simulink model "TST_StSys_StrtRmp"  (R2016b)
settings: Solver=FixedStepDiscrete  StartTime=0.0  StopTime=simTime  FixedStep=sampleTime  RelTol=1e-3
values from neighbouring files (symbols this model uses):
  testCase = 1    [initTST_StSys_StrtRmp_001.m]
libraries: simulink x3, UnitTest_Lib x1
settings Model: Creator=zhengjinyan  LastModifiedBy=zhengjinyan
settings DebuggingCC: SignalRangeChecking=error

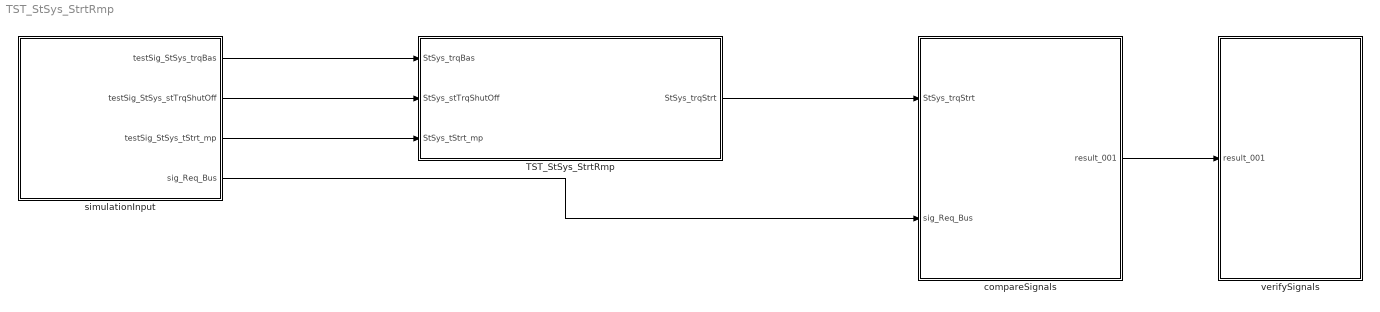
== system TST_StSys_StrtRmp ==
  TST_StSys_StrtRmp : Subsystem
  compareSignals : Subsystem
  simulationInput : Subsystem
  verifySignals : Subsystem
  wires:
  simulationInput/1(testSig_StSys_trqBas) -> TST_StSys_StrtRmp/1(StSys_trqBas)
  simulationInput/2(testSig_StSys_stTrqShutOff) -> TST_StSys_StrtRmp/2(StSys_stTrqShutOff)
  simulationInput/3(testSig_StSys_tStrt_mp) -> TST_StSys_StrtRmp/3(StSys_tStrt_mp)
  TST_StSys_StrtRmp/1(StSys_trqStrt) -> compareSignals/1(StSys_trqStrt)
  simulationInput/4(sig_Req_Bus) -> compareSignals/2(sig_Req_Bus)
  compareSignals/1(result_001) -> verifySignals/1(result_001)

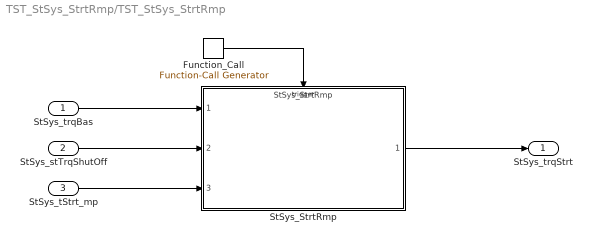
== system TST_StSys_StrtRmp/TST_StSys_StrtRmp ==
  StSys_trqBas : Inport
  StSys_stTrqShutOff : Inport  Port=2
  StSys_tStrt_mp : Inport  Port=3
  Function_Call : simulink/Ports & Subsystems/Function-Call Generator  sample_time=sampleTime  numberOfIterations=1
  StSys_StrtRmp : ModelReference  ModelNameDialog=StSys_StrtRmp  SimulationMode=Normal  ModelReferenceVersion=1.51  TriggerPortName=function  TriggerPortTriggerType=function-call  TriggerPortStatesWhenEnabling=held
  StSys_trqStrt : Outport
  wires:
  Function_Call/1 -> StSys_StrtRmp/Trigger
  StSys_trqBas/1 -> StSys_StrtRmp/1
  StSys_stTrqShutOff/1 -> StSys_StrtRmp/2
  StSys_tStrt_mp/1 -> StSys_StrtRmp/3
  StSys_StrtRmp/1 -> StSys_trqStrt/1

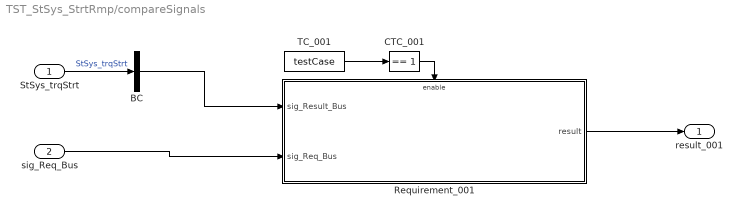
== system TST_StSys_StrtRmp/compareSignals ==
  StSys_trqStrt : Inport
  sig_Req_Bus : Inport  Port=2
  BC : BusCreator  Inputs=1
  CTC_001 : simulink/Logic and Bit Operations/Compare To Constant  relop===  const=1  OutDataTypeStr=boolean
  Requirement_001 : Subsystem
  TC_001 : Constant  Value=testCase
  result_001 : Outport
  wires:
  StSys_trqStrt/1 -> BC/1  "StSys_trqStrt"
  TC_001/1 -> CTC_001/1
  CTC_001/1 -> Requirement_001/Enable
  sig_Req_Bus/1 -> Requirement_001/2(sig_Req_Bus)
  BC/1 -> Requirement_001/1(sig_Result_Bus)
  Requirement_001/1(result) -> result_001/1

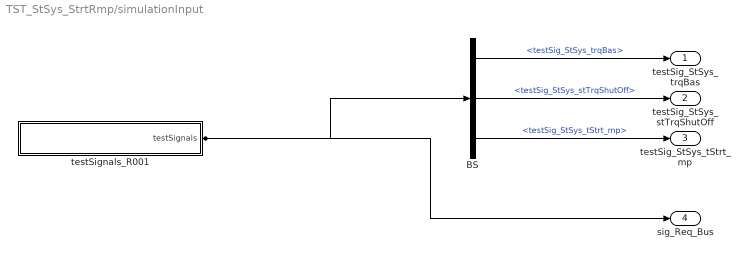
== system TST_StSys_StrtRmp/simulationInput ==
  BS : BusSelector  OutputSignals=testSig_StSys_trqBas,testSig_StSys_stTrqShutOff,testSig_StSys_tStrt_mp
  testSignals_R001 : Subsystem
  testSig_StSys_trqBas : Outport
  testSig_StSys_stTrqShutOff : Outport  Port=2
  testSig_StSys_tStrt_mp : Outport  Port=3
  sig_Req_Bus : Outport  Port=4
  wires:
  BS/1 -> testSig_StSys_trqBas/1  "<testSig_StSys_trqBas>"
  BS/2 -> testSig_StSys_stTrqShutOff/1  "<testSig_StSys_stTrqShutOff>"
  BS/3 -> testSig_StSys_tStrt_mp/1  "<testSig_StSys_tStrt_mp>"
  testSignals_R001/1(testSignals) -> BS/1, sig_Req_Bus/1

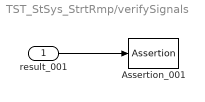
== system TST_StSys_StrtRmp/verifySignals ==
  result_001 : Inport
  Assertion_001 : Assertion  Enabled=off
  wires:
  result_001/1 -> Assertion_001/1

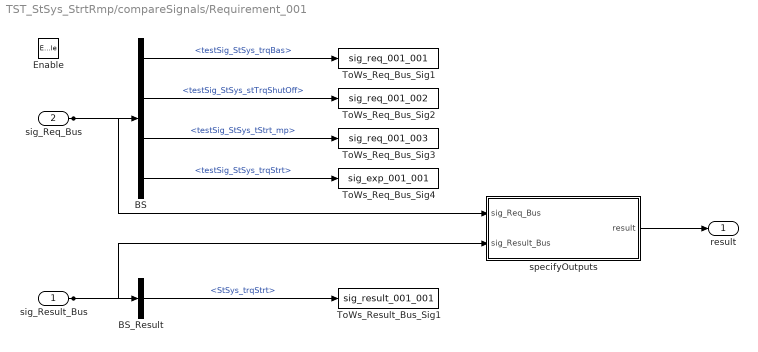
== system TST_StSys_StrtRmp/compareSignals/Requirement_001 ==
  sig_Result_Bus : Inport
  sig_Req_Bus : Inport  Port=2
  Enable : EnablePort
  BS : BusSelector  OutputSignals=testSig_StSys_trqBas,testSig_StSys_stTrqShutOff,testSig_StSys_tStrt_mp,testSig_StSys_trqStrt
  BS_Result : BusSelector  OutputSignals=StSys_trqStrt
  ToWs_Req_Bus_Sig1 : ToWorkspace  VariableName=sig_req_001_001  SaveFormat=Structure With Time
  ToWs_Req_Bus_Sig2 : ToWorkspace  VariableName=sig_req_001_002  SaveFormat=Structure With Time
  ToWs_Req_Bus_Sig3 : ToWorkspace  VariableName=sig_req_001_003  SaveFormat=Structure With Time
  ToWs_Req_Bus_Sig4 : ToWorkspace  VariableName=sig_exp_001_001  SaveFormat=Structure With Time
  ToWs_Result_Bus_Sig1 : ToWorkspace  VariableName=sig_result_001_001  SaveFormat=Structure With Time
  specifyOutputs : Subsystem
  result : Outport
  wires:
  sig_Req_Bus/1 -> BS/1, specifyOutputs/1(sig_Req_Bus)
  BS/1 -> ToWs_Req_Bus_Sig1/1  "<testSig_StSys_trqBas>"
  BS/2 -> ToWs_Req_Bus_Sig2/1  "<testSig_StSys_stTrqShutOff>"
  BS/3 -> ToWs_Req_Bus_Sig3/1  "<testSig_StSys_tStrt_mp>"
  BS/4 -> ToWs_Req_Bus_Sig4/1  "<testSig_StSys_trqStrt>"
  sig_Result_Bus/1 -> BS_Result/1, specifyOutputs/2(sig_Result_Bus)
  BS_Result/1 -> ToWs_Result_Bus_Sig1/1  "<StSys_trqStrt>"
  specifyOutputs/1(result) -> result/1

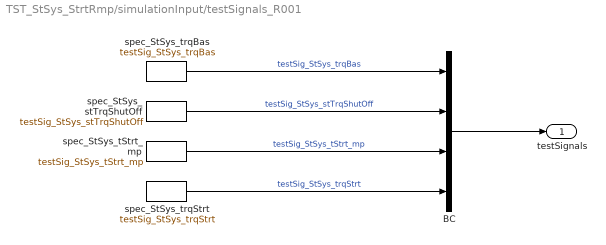
== system TST_StSys_StrtRmp/simulationInput/testSignals_R001 ==
  BC : BusCreator  Inputs=4
  spec_StSys_stTrqShutOff : FromWorkspace  VariableName=testSig_StSys_stTrqShutOff  Interpolate=off  OutputAfterFinalValue=Holding final value
  spec_StSys_tStrt_mp : FromWorkspace  VariableName=testSig_StSys_tStrt_mp  Interpolate=off  OutputAfterFinalValue=Holding final value
  spec_StSys_trqBas : FromWorkspace  VariableName=testSig_StSys_trqBas  Interpolate=off  OutputAfterFinalValue=Holding final value
  spec_StSys_trqStrt : FromWorkspace  VariableName=testSig_StSys_trqStrt  Interpolate=off  OutputAfterFinalValue=Holding final value
  testSignals : Outport
  wires:
  BC/1 -> testSignals/1
  spec_StSys_trqBas/1 -> BC/1  "testSig_StSys_trqBas"
  spec_StSys_stTrqShutOff/1 -> BC/2  "testSig_StSys_stTrqShutOff"
  spec_StSys_tStrt_mp/1 -> BC/3  "testSig_StSys_tStrt_mp"
  spec_StSys_trqStrt/1 -> BC/4  "testSig_StSys_trqStrt"

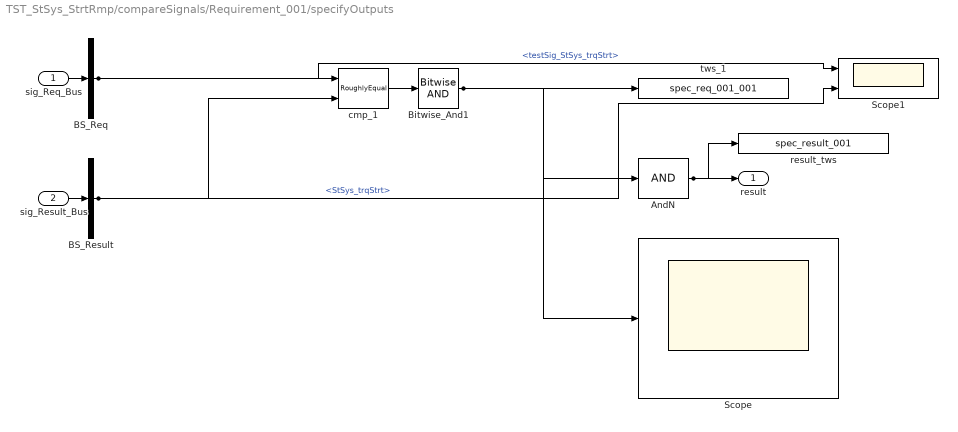
== system TST_StSys_StrtRmp/compareSignals/Requirement_001/specifyOutputs ==
  sig_Req_Bus : Inport
  sig_Result_Bus : Inport  Port=2
  AndN : Logic  Inputs=1
  BS_Req : BusSelector  OutputSignals=testSig_StSys_trqStrt
  BS_Result : BusSelector  OutputSignals=StSys_trqStrt
  Bitwise_And1 : simulink/Logic and Bit Operations/Bitwise Operator  logicop=AND  UseBitMask=off  BitMask=bin2dec('11011001')  BitMaskRealWorld=Stored Integer
  Scope : Scope
  Scope1 : Scope  NumInputPorts=2
  cmp_1 : UnitTest_Lib/RoughlyEqual  slope=0.1
  result_tws : ToWorkspace  VariableName=spec_result_001
  tws_1 : ToWorkspace  VariableName=spec_req_001_001
  result : Outport
  wires:
  sig_Req_Bus/1 -> BS_Req/1
  sig_Result_Bus/1 -> BS_Result/1
  AndN/1 -> result/1, result_tws/1
  BS_Req/1 -> cmp_1/1, Scope1/1  "<testSig_StSys_trqStrt>"
  BS_Result/1 -> cmp_1/2, Scope1/2  "<StSys_trqStrt>"
  cmp_1/1 -> Bitwise_And1/1
  Bitwise_And1/1 -> tws_1/1, AndN/1, Scope/1
